simulink model "test_pid_tv"  (R2024b)
settings: Solver=VariableStepAuto  StartTime=0.0  StopTime=10.0  RelTol=1e-3
libraries: simulink_extras x1, slpidlib x1
settings Model: Creator=lukec  LastModifiedBy=lukec

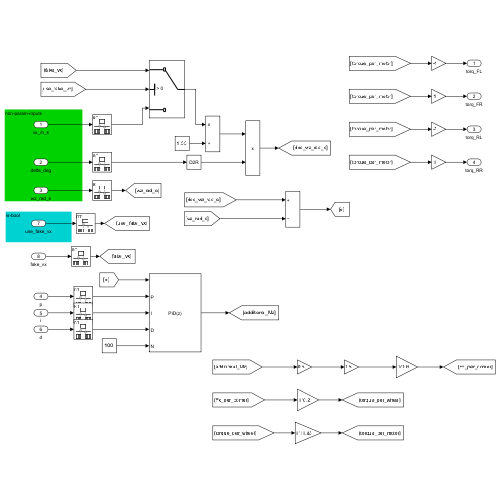
[thumbnail: Simulink's stored preview of the top-level diagram]
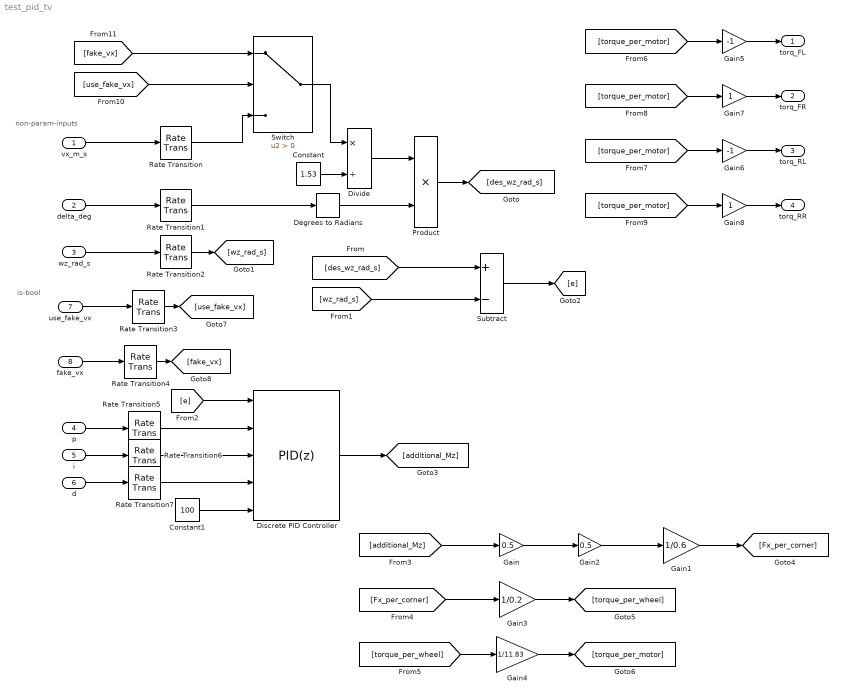
== system test_pid_tv ==
  note: non-param-inputs
  note: is-bool
  vx_m_s : Inport
  delta_deg : Inport  Port=2
  wz_rad_s : Inport  Port=3
  p : Inport  Port=4
  i : Inport  Port=5
  d : Inport  Port=6
  use_fake_vx : Inport  Port=7
  fake_vx : Inport  Port=8
  Constant : Constant  Value=1.53
  Constant1 : Constant  Value=100
  Degrees to Radians : simulink_extras/Transformations/Degrees to Radians
  Discrete PID Controller : slpidlib/PID Controller  Controller=PID  Form=Parallel  TimeDomain=Discrete-time  UseExternalTs=off  SampleTime=-1  IntegratorMethod=Forward Euler  FilterMethod=Forward Euler  ControllerParametersSource=external  P=1  I=1  UseKiTs=off  D=0  UseExternalDerivativeSource=off  N=100  UseFilter=on  TunerSelectOption=Transfer Function Based (PID Tuner App)  InitialConditionSource=internal  InitialConditionForIntegrator=0  InitialConditionForFilter=0  DifferentiatorICPrevScaledInput=0  ExternalReset=none  TrackingMode=off  Kt=1  LimitOutput=off  SatLimitsSource=internal  UpperSaturationLimit=inf  LowerSaturationLimit=-inf  LinearizeAsGain=off  AntiWindupMode=none  Kb=1  LimitIntegrator=off  UpperIntegratorSaturationLimit=inf  LowerIntegratorSaturationLimit=-inf  POutMin=[]  POutMax=[]  IOutMin=[]  IOutMax=[]  DOutMin=[]  DOutMax=[]  NOutMin=[]  NOutMax=[]  SumOutMin=[]  SumOutMax=[]  SaturationOutMin=[]  SaturationOutMax=[]  PParamMin=[]  PParamMax=[]  IParamMin=[]  IParamMax=[]  DParamMin=[]  DParamMax=[]  NParamMin=[]  NParamMax=[]  KbParamMin=[]  KbParamMax=[]  KtParamMin=[]  KtParamMax=[]  KbOutMin=[]  KbOutMax=[]  KtOutMin=[]  KtOutMax=[]  IntegratorOutMin=[]  IntegratorOutMax=[]  FilterOutMin=[]  FilterOutMax=[]  SumI1OutMin=[]  SumI1OutMax=[]  SumI2OutMin=[]  SumI2OutMax=[]  SumI3OutMin=[]  SumI3OutMax=[]  SumI4OutMin=[]  SumI4OutMax=[]  SumDOutMin=[]  SumDOutMax=[]  DifferentiatorOutMin=[]  DifferentiatorOutMax=[]  FilterDiffOutCoefMin=[]  FilterDiffOutCoefMax=[]  ReciprocalOutMin=[]  ReciprocalOutMax=[]  SumDenOutMin=[]  SumDenOutMax=[]  SumNumOutMin=[]  SumNumOutMax=[]  DivideOutMin=[]  DivideOutMax=[]  UdiffTsProdOutMin=[]  UdiffTsProdOutMax=[]  NTsProdOutMin=[]  NTsProdOutMax=[]  UintegralTsProdOutMin=[]  UintegralTsProdOutMax=[]  UngainTsProdOutMin=[]  UngainTsProdOutMax=[]  ClampingZeroOutDataTypeStr=Inherit: Inherit via back propagation  ClampingZeroOutMin=[]  ClampingZeroOutMax=[]  FilterDenConstantOutDataTypeStr=Inherit: Inherit via back propagation  FilterDenConstantOutMin=[]  FilterDenConstantOutMax=[]  PCopyOutDataTypeStr=Inherit: Inherit via back propagation  PCopyOutMin=[]  PCopyOutMax=[]  NCopyOutDataTypeStr=Inherit: Inherit via back propagation  NCopyOutMin=[]  NCopyOutMax=[]  IntegratorContinuousStateAttributes=''  IntegratorStateMustResolveToSignalObject=off  IntegratorRTWStateStorageClass=Auto  FilterContinuousStateAttributes=''  FilterStateMustResolveToSignalObject=off  FilterRTWStateStorageClass=Auto  ParallelPVariant=ExternalParameters  IdealPVariant=Disabled  IVariant=ExternalParameters  DVariant=ExternalParameters  IntegratorVariant=Discrete  SatVariant=Disabled  AWVariant=Passthrough  PCopyVariant=Disabled  TRVariant=Disabled  FdbkBlocksVariant=Forward  IdealPFdbkVariant=Disabled  SatFdbkVariant=Disabled  DerivativeFilterVariant=ForwardEulerFilter  NVariant=ExternalParameters  NCopyVariant=Disabled  FilterICVariant=InternalICsFilter  IntegratorICVariant=InternalICs  ExternalResetVariant=Disabled  TRSumVariant=Passthrough  SumFdbkVariant=Disabled  SumVariant=Sum_PID  TsampFilterVariant=InternalTs  TsampNgainVariant=Passthrough  TsampIntegralVariant=Disabled_SignalSpec  ExternalSaturationOutDataTypeStr=Inherit: Same as second input  DerivativeSourceVariant=ErrorSignal  PreIntVariant=InternalPreInt
      settings: LibrarySourceBlock=simulink/Discrete/Discrete PID Controller
  Divide : Product  Inputs=*/
  Gain : Gain  Gain=0.5
  Gain1 : Gain  Gain=1/0.6
  Gain2 : Gain  Gain=0.5
  Gain3 : Gain  Gain=1/0.2
  Gain4 : Gain  Gain=1/11.83
  Gain5 : Gain  Gain=-1
  Gain6 : Gain  Gain=-1
  Gain7 : Gain
  Gain8 : Gain
  Product : Product
  Rate Transition{,1..7} (8 alike) : RateTransition  OutPortSampleTime=0.01
  Subtract : Sum  Inputs=+-
  Switch : Switch  Criteria=u2 > Threshold  SaturateOnIntegerOverflow=off  InputSameDT=off
  torq_FL : Outport
  torq_FR : Outport  Port=2
  torq_RL : Outport  Port=3
  torq_RR : Outport  Port=4
  wires:
  Constant/1 -> Divide/2
  Divide/1 -> Product/1
  delta_deg/1 -> Rate Transition1/1
  Degrees to Radians/1 -> Product/2
  Product/1 -> [des_wz_rad_s]
  [des_wz_rad_s] -> Subtract/1
  wz_rad_s/1 -> Rate Transition2/1
  [wz_rad_s] -> Subtract/2
  Subtract/1 -> [e]
  [e] -> Discrete PID Controller/1
  p/1 -> Rate Transition5/1
  i/1 -> Rate Transition6/1
  d/1 -> Rate Transition7/1
  Constant1/1 -> Discrete PID Controller/5
  Discrete PID Controller/1 -> [additional_Mz]
  [additional_Mz] -> Gain/1
  Gain/1 -> Gain2/1
  Gain2/1 -> Gain1/1
  Gain1/1 -> [Fx_per_corner]
  [Fx_per_corner] -> Gain3/1
  Gain3/1 -> [torque_per_wheel]
  [torque_per_wheel] -> Gain4/1
  Gain4/1 -> [torque_per_motor]
  [torque_per_motor] -> Gain5/1
  [torque_per_motor] -> Gain6/1
  Gain5/1 -> torq_FL/1
  [torque_per_motor] -> Gain7/1
  [torque_per_motor] -> Gain8/1
  Gain6/1 -> torq_RL/1
  Gain7/1 -> torq_FR/1
  Gain8/1 -> torq_RR/1
  use_fake_vx/1 -> Rate Transition3/1
  fake_vx/1 -> Rate Transition4/1
  [use_fake_vx] -> Switch/2
  [fake_vx] -> Switch/1
  vx_m_s/1 -> Rate Transition/1
  Switch/1 -> Divide/1
  Rate Transition/1 -> Switch/3
  Rate Transition1/1 -> Degrees to Radians/1
  Rate Transition2/1 -> [wz_rad_s]
  Rate Transition3/1 -> [use_fake_vx]
  Rate Transition4/1 -> [fake_vx]
  Rate Transition5/1 -> Discrete PID Controller/2
  Rate Transition6/1 -> Discrete PID Controller/3
  Rate Transition7/1 -> Discrete PID Controller/4
